simulink model "PID_Controller"  (R2020b)
settings: Solver=VariableStepAuto  StartTime=0.0  StopTime=120  RelTol=1e-3
model mask{Kd=0, Ki=0, Kp=0}
model workspace (MAT data in the model file):
  Kd = 484.0516
  Ki = 83.0917
  Kp = 495.0505
values from neighbouring files (symbols this model uses):
  N = 100000.0    [Data.sldd]
settings Model: DataDictionary=Data.sldd  ParameterArgumentNames=Kd,Ki,Kp  Creator=vigne  LastModifiedBy=vigne
settings DataIOCC: SaveOutput=off  SaveTime=off

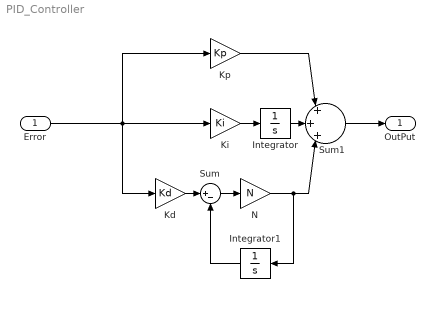
== system PID_Controller ==
  Error : Inport  OutDataTypeStr=double  PortDimensions=1
  Integrator : Integrator
  Integrator1 : Integrator
  Kd : Gain  Gain=Kd
  Ki : Gain  Gain=Ki
  Kp : Gain  Gain=Kp
  N : Gain  Gain=N
  Sum : Sum  Inputs=|+-
  Sum1 : Sum  Inputs=|+|+|+|
  OutPut : Outport  OutDataTypeStr=double  PortDimensions=1  SampleTime=0
  wires:
  Ki/1 -> Integrator/1
  Kp/1 -> Sum1/1
  Error/1 -> Ki/1, Kp/1, Kd/1
  N/1 -> Integrator1/1, Sum1/3
  Integrator/1 -> Sum1/2
  Sum1/1 -> OutPut/1
  Kd/1 -> Sum/1
  Sum/1 -> N/1
  Integrator1/1 -> Sum/2
